simulink model "PubIfDecisionTOS_MDL"  (R2020b)
settings: configuration reference "DspaceConfig" (kept outside this file)
PostLoadFcn:
  | if any(exist('dsrtsu_mdlpostloadfcn', 'file') ~= 0), dsrtsu_mdlpostloadfcn('Execute', bdroot); end
InitFcn:
  | , if any(exist('dsmpb_private', 'file') ~= 0), dsmpb_private('dsmpb_mdlclblib', 'Init', bdroot); end,
undefined symbols (not defined in the file or in its folder): C_TOS_ACCEgoRAxletoFbumplength_m, C_TOS_ACCTargetFront_Flag, C_TOS_AEBJAPedObjDxThre_Val, C_TOS_AEBJAPedObjDyThre_Val, C_TOS_AEBJATargetSize_Val, C_TOS_AEBJAVehObjDxThre_Val, C_TOS_AEBJAVehObjDyThre_Val, C_TOS_AEBJuncPedTargetSize_Val, C_TOS_AEBLatObjDxThre_Val, C_TOS_AEBLatPedDyThre_Val, C_TOS_AEBLatTargetSize_Val, C_TOS_AEBLongTargetInEgoFront_Flag, C_TOS_axAbsGround_Parameter, C_TOS_CameraConfirmedFlag, C_TOS_CNsubjWidth, C_TOS_CurrentLaneCoreMinWidth_Val, C_TOS_CutInProb_Val_Zero, C_TOS_CutOutProb_Val_Zero, C_TOS_D2R_Val, C_TOS_DefaultValueObjectToCenterLine_dy, C_TOS_EgoCarWidth_Val, C_TOS_EgoDxRefPoint_m, C_TOS_EgoRAxletoFbumplength_m, C_TOS_HalfWidthVehicle_Con, C_TOS_HWA_CurrentLaneFlag, C_TOS_HWA_LeftLaneFlag, C_TOS_HWA_MovingDir_Vaild, C_TOS_HWA_MovState_Vaild, C_TOS_HWA_RightLaneFlag, C_TOS_LaneLineCourseErrorFront, C_TOS_LaneLineCourseErrorRear, C_TOS_MotorbikeDefaultWidth_m, C_TOS_NumberOfEffectiveTargets, C_TOS_Obj_Age_Val, C_TOS_Objdx_Constraint_Val, C_TOS_ObjectDefaultWidth_m, C_TOS_ObjInCurrentLane_Val, C_TOS_ObjInCurrentLaneValid, C_TOS_ObjInLeftLaneValid, C_TOS_ObjInRightLaneValid, C_TOS_ObjNotInCurrentLane_Val, C_TOS_ObjNotREElementType, C_TOS_ObjPredictDis_dy_ConstantVal_Zeros, C_TOS_ObjToCenterLine_ConstantVal_Zeros, C_TOS_OFMObjIDInvilad_Val, C_TOS_PIL_LatDisCons_Val_zero, C_TOS_PIL_ObjectCutInFlag_b, C_TOS_PIL_ObjectCutOutFlag_b, C_TOS_PIL_ObjLaneProb_al_Val, C_TOS_PP_ObjFusType_FC_Confirm_b, C_TOS_PP_ObjFusType_FC_FR_Confirm_b, C_TOS_PP_ObjFusType_FR_Confirm_b, C_TOS_RE_80BoolDefault_Val, C_TOS_RE_80Single181Default_Val, C_TOS_RE_80Single255Default_Val, C_TOS_RE_80Uint8Default_Val, C_TOS_RE_D2R, C_TOS_RE_D_180_Val, C_TOS_RE_InvalidObjectID_Val, C_TOS_RE_InvalidTargetChainDir_Val ... (+142)
libraries: simulink x1650, TOS_LIB x361, canfdmsglib x14
(part 34 of 69)

== system PubIfDecisionTOS_MDL/TOS_20201112/TOS_2012080320/PP1128/AAT-AdditionalAttributes/PP_ObjectToCenterLine_dy/PP_EgoVeh_Object_ToCenterLine/PP_ObjectToCenterLine/PP_ObjectToCenterLine_/line05_dy ==
  Object_DX : Inport
  line05_C0 : Inport  Port=2
  line05_C1 : Inport  Port=3
  line05_C2 : Inport  Port=4
  line05_C3 : Inport  Port=5
  Add : Sum
  Add1 : Sum
  Add3 : Sum
  Constant1 : Constant  Value=3  OutDataTypeStr=single
  Math Function1 : Math  Operator=pow  SignedPower=on  SaturateOnIntegerOverflow=on
  Product : Product
  Product1 : Product
  Product2 : Product
  Square : Math  Operator=square  SignedPower=on  SaturateOnIntegerOverflow=on
  line05_dy : Outport
  wires:
  line05_C1/1 -> Product1/2
  line05_C3/1 -> Product2/2
  Add3/1 -> line05_dy/1
  Add/1 -> Add3/1
  Constant1/1 -> Math Function1/2
  Product1/1 -> Add1/2
  Product2/1 -> Add3/2
  Math Function1/1 -> Product2/1
  Object_DX/1 -> Math Function1/1, Square/1, Product1/1
  Square/1 -> Product/1
  line05_C2/1 -> Product/2
  Product/1 -> Add/2
  line05_C0/1 -> Add1/1
  Add1/1 -> Add/1

== system PubIfDecisionTOS_MDL/TOS_20201112/TOS_2012080320/PP1128/AAT-AdditionalAttributes/PP_ObjectToCenterLine_dy/PP_EgoVeh_Object_ToCenterLine/PP_ObjectToCenterLine/PP_ObjectToCenterLine_/line06_DisJudge ==
  Object_DX : Inport
  line06_dDisStart : Inport  Port=2
  line06_dDisEnd : Inport  Port=3
  Logical Operator : Logic  AllPortsSameDT=off  OutDataTypeStr=boolean
  Relational Operator : RelationalOperator  OutDataTypeStr=boolean  RndMeth=Nearest
  Relational Operator1 : RelationalOperator  Operator=<  OutDataTypeStr=boolean  RndMeth=Nearest
  line06_DisJudge : Outport
  wires:
  Logical Operator/1 -> line06_DisJudge/1
  Relational Operator1/1 -> Logical Operator/2
  Relational Operator/1 -> Logical Operator/1
  Object_DX/1 -> Relational Operator/1, Relational Operator1/1
  line06_dDisStart/1 -> Relational Operator/2
  line06_dDisEnd/1 -> Relational Operator1/2

== system PubIfDecisionTOS_MDL/TOS_20201112/TOS_2012080320/PP1128/AAT-AdditionalAttributes/PP_ObjectToCenterLine_dy/PP_EgoVeh_Object_ToCenterLine/PP_ObjectToCenterLine/PP_ObjectToCenterLine_/line06_dy ==
  Object_DX : Inport
  line06_C0 : Inport  Port=2
  line06_C1 : Inport  Port=3
  line06_C2 : Inport  Port=4
  line6_C3 : Inport  Port=5
  Add : Sum
  Add1 : Sum
  Add3 : Sum
  Constant1 : Constant  Value=3  OutDataTypeStr=single
  Math Function1 : Math  Operator=pow  SignedPower=on  SaturateOnIntegerOverflow=on
  Product : Product
  Product1 : Product
  Product2 : Product
  Square : Math  Operator=square  SignedPower=on  SaturateOnIntegerOverflow=on
  line6_dy : Outport
  wires:
  Add1/1 -> Add/1
  line06_C0/1 -> Add1/1
  Product/1 -> Add/2
  line06_C2/1 -> Product/2
  Square/1 -> Product/1
  Object_DX/1 -> Product1/1, Square/1, Math Function1/1
  Math Function1/1 -> Product2/1
  Product2/1 -> Add3/2
  Product1/1 -> Add1/2
  Constant1/1 -> Math Function1/2
  Add/1 -> Add3/1
  Add3/1 -> line6_dy/1
  line6_C3/1 -> Product2/2
  line06_C1/1 -> Product1/2

== system PubIfDecisionTOS_MDL/TOS_20201112/TOS_2012080320/PP1128/AAT-AdditionalAttributes/PP_ObjectToCenterLine_dy/PP_ObjectToCenterLine_vyc/PP_ObjectToCenterLine_vyc_Filt/ObjectToCenterLine_vyc/ObjectToCenterLine_vyc_Filt ==
  ObjectID_Filt_K1 : Inport
  PP_ObjectToCenterLine_vyc_Filt_K1 : Inport  Port=2  OutDataTypeStr=single
  PP_ObjectToCenterLine_vyc : Inport  Port=3  OutDataTypeStr=single
  Object_ID : Inport  Port=4  OutDataTypeStr=uint8
  Object_Age : Inport  Port=5
  TOS_OFMObjValid_Flag : Inport  Port=6
  Action Port : ActionPort  ActionPortLabel=else
  Constant1 : Constant  Value=C_TOS_NumberOfEffectiveTargets  OutDataTypeStr=int32
      settings: AttributesFormatString=C_TOS_NumberOfEffectiveTargets = 80
  Constant2 : Constant  Value=0.2  OutDataTypeStr=single
      settings: AttributesFormatString=P_TOS_PIL_ObjectToCenterLine_dy_CutInDeclineLimit = 0.1
  Constant8 : Constant  Value=0.35  OutDataTypeStr=single
      settings: AttributesFormatString=P_TOS_PIL_ObjectToCenterLine_dy_CutInUpperLimit = 0.5
  ObjectToCenterLine_vyc_Filt : MATLAB Function  TreatAsAtomicUnit=on
  Terminator : Terminator
  Obj_ID : Outport
  PP_ObjectToCenterLine_vyc_Filt : Outport  Port=2  OutDataTypeStr=single
  wires:
  TOS_OFMObjValid_Flag/1 -> ObjectToCenterLine_vyc_Filt/5(TOS_OFMObjValid_Flag)
  Object_Age/1 -> Terminator/1
  PP_ObjectToCenterLine_vyc_Filt_K1/1 -> ObjectToCenterLine_vyc_Filt/2(ObjectToCenterLine_dy_Filt_K1)
  Object_ID/1 -> Obj_ID/1, ObjectToCenterLine_vyc_Filt/4(Object_ID)
  ObjectID_Filt_K1/1 -> ObjectToCenterLine_vyc_Filt/1(ObjectID_Filt_K1)
  Constant2/1 -> ObjectToCenterLine_vyc_Filt/7(P_TOS_PIL_ObjectToCenterLine_dy_CutInDeclineLimit)
  Constant1/1 -> ObjectToCenterLine_vyc_Filt/8(Iterator_Num)
  PP_ObjectToCenterLine_vyc/1 -> ObjectToCenterLine_vyc_Filt/3(ObjectToCenterLine_dy)
  Constant8/1 -> ObjectToCenterLine_vyc_Filt/6(P_TOS_PIL_ObjectToCenterLine_dy_CutInUpperLimit)
  ObjectToCenterLine_vyc_Filt/1(ObjectToCenterLine_dy_Filt) -> PP_ObjectToCenterLine_vyc_Filt/1

== system PubIfDecisionTOS_MDL/TOS_20201112/TOS_2012080320/PP1128/AAT-AdditionalAttributes/PP_ObjectToCenterLine_dy/PP_ObjectToCenterLine_vyc/PP_ObjectToCenterLine_vyc_Filt/ObjectToCenterLine_vyc/ObjectToCenterLine_vyc_FiltDefault ==
  Action Port : ActionPort  ActionPortLabel=if(u1 ~= 0)
  Constant : Constant  Value=0  OutDataTypeStr=uint8
  Constant1 : Constant  Value=255  OutDataTypeStr=single
  Obj_ID : Outport
  ObjectToCenterLine_dy_Filt : Outport  Port=2  OutDataTypeStr=single
  wires:
  Constant1/1 -> ObjectToCenterLine_dy_Filt/1
  Constant/1 -> Obj_ID/1

== system PubIfDecisionTOS_MDL/TOS_20201112/TOS_2012080320/PP1128/AAT-AdditionalAttributes/RoadEdge/RE_2020_12_07/RoadEdge_V2/RoadEdgeElementFinalJudge/EgoLeft_RoadEdgeElementsFinalJudge ==
  RE_EgoLeftEdgeGroupChainElementCount : Inport  OutDataTypeStr=uint8  BusOutputAsStruct=on
  RE_EgoLeft_3TargetTheta : Inport  Port=2  OutDataTypeStr=single  BusOutputAsStruct=on
  RE_EgoLeft_2TargetTheta : Inport  Port=3  OutDataTypeStr=single  BusOutputAsStruct=on
  RE_EgoLeft_StillObjSortIndex : Inport  Port=4  OutDataTypeStr=uint8  BusOutputAsStruct=on
  vxvRefMs : Inport  Port=5  OutDataTypeStr=single  PortDimensions=1  BusOutputAsStruct=on
  Object_Dx : Inport  Port=6  OutDataTypeStr=single  BusOutputAsStruct=on
  Object_Dy : Inport  Port=7  OutDataTypeStr=single  BusOutputAsStruct=on
  Object_ID : Inport  Port=8  OutDataTypeStr=uint8  BusOutputAsStruct=on
  RE_EdgeElementID_K1 : Inport  Port=9
  Dy_Filter : Subsystem
  For Each Subsystem : Subsystem  TreatAsAtomicUnit=on
  RoadEdgeElementFinalJudge : Stateflow chart  TreatAsAtomicUnit=on
  Unit Delay{,1..3} (4 alike) : UnitDelay  SampleTime=-1  HasFrameUpgradeWarning=on
  RE_EgoLeftEdgeElementFlag : Outport
  RE_EgoLeftEdgeElementType : Outport  Port=2
  StillTarget34_13_Theta_ALL : Outport  Port=3
  RE_EgoLeftEdgeElementID : Outport  Port=4
  EdgeGroupChainElementCount_OFM : Outport  Port=5
  wires:
  RE_EgoLeftEdgeGroupChainElementCount/1 -> RoadEdgeElementFinalJudge/2(EdgeGroupChainElementCount)
  RE_EgoLeft_3TargetTheta/1 -> RoadEdgeElementFinalJudge/3(RE_3TargetTheta)
  RE_EgoLeft_2TargetTheta/1 -> RoadEdgeElementFinalJudge/4(RE_2TargetTheta)
  RE_EgoLeft_StillObjSortIndex/1 -> RoadEdgeElementFinalJudge/5(RE_StillObjectSortIndex), Unit Delay2/1
  Object_Dx/1 -> RoadEdgeElementFinalJudge/8(Object_Dx)
  vxvRefMs/1 -> RoadEdgeElementFinalJudge/7(Ego_Vxv)
  Object_ID/1 -> Dy_Filter/4(Object_ID), RoadEdgeElementFinalJudge/10(Object_ID)
  RoadEdgeElementFinalJudge/1(RoadEdgeElementFlag) -> Unit Delay/1, RE_EgoLeftEdgeElementFlag/1  "EdgeElementFlag"
  RoadEdgeElementFinalJudge/2(RE_EdgeElementType) -> RE_EgoLeftEdgeElementType/1  "EdgeElementType"
  RoadEdgeElementFinalJudge/3(StillTarget34_13_Theta_ALL) -> StillTarget34_13_Theta_ALL/1  "StillTarget34_13_Theta_ALL"
  RoadEdgeElementFinalJudge/4(RE_EdgeElementID) -> RE_EgoLeftEdgeElementID/1  "RE_EgoLeftEdgeElementID"
  RoadEdgeElementFinalJudge/5(StillTarget13_Theta_ALL) -> Unit Delay1/1
  Unit Delay1/1 -> RoadEdgeElementFinalJudge/11(RE_13TargetTheta_ALL)
  Unit Delay2/1 -> RoadEdgeElementFinalJudge/6(RE_StillObjectSortIndex_K1)
  Object_Dy/1 -> Dy_Filter/1(Object_Dy), Unit Delay3/1
  Unit Delay3/1 -> Dy_Filter/2(Object_Dy_K1)
  Dy_Filter/1(Object_DyFilter) -> RoadEdgeElementFinalJudge/9(Object_Dy)
  For Each Subsystem/1(RE_4StepEdgeElementFlag) -> RoadEdgeElementFinalJudge/1(RE_4StepEdgeElementFlag)
  Unit Delay/1 -> For Each Subsystem/1(RE_EdgeElementFlag)
  RoadEdgeElementFinalJudge/10(EdgeGroupChainElementCount_OFM) -> EdgeGroupChainElementCount_OFM/1
  RE_EdgeElementID_K1/1 -> Dy_Filter/3(RE_EdgeElementID_K1)

== system PubIfDecisionTOS_MDL/TOS_20201112/TOS_2012080320/PP1128/AAT-AdditionalAttributes/RoadEdge/RE_2020_12_07/RoadEdge_V2/RoadEdgeElementFinalJudge/EgoRight_RoadEdgeElementsFinalJudge ==
  note: 13_Theta
  note: StillTarget34_13_Theta_ALL
  note: StillObjSortIndex
  note: 2TargetTheta
  note: 3TargetTheta
  note: RE_EgoRightEdgeGroupChainElementCount
  note: StillTarget13_Theta_OFM
  note: StillTarget34_13_Theta_OFM
  note: RE_EdgeElementID
  note: StillTarget3Theta_OFM
  note: StillTarget2Theta_OFM
  RE_EgoRightEdgeGroupChainElementCount : Inport  OutDataTypeStr=uint8  BusOutputAsStruct=on
  RE_EgoRight_3TargetTheta : Inport  Port=2  OutDataTypeStr=single  BusOutputAsStruct=on
  RE_EgoRight_2TargetTheta : Inport  Port=3  OutDataTypeStr=single  BusOutputAsStruct=on
  RE_EgoRight_StillObjSortIndex : Inport  Port=4  OutDataTypeStr=uint8  BusOutputAsStruct=on
  vxvRefMs : Inport  Port=5  OutDataTypeStr=single  PortDimensions=1  BusOutputAsStruct=on
  Object_Dx : Inport  Port=6  OutDataTypeStr=single  BusOutputAsStruct=on
  Object_Dy : Inport  Port=7  OutDataTypeStr=single  BusOutputAsStruct=on
  Object_ID : Inport  Port=8  OutDataTypeStr=uint8  BusOutputAsStruct=on
  RE_EdgeElementID_K1 : Inport  Port=9
  Display{1..12} (12 alike) : Display
  Dy_Filter : Subsystem
  For Each Subsystem : Subsystem  TreatAsAtomicUnit=on
  RoadEdgeElementFinalJudge : Stateflow chart  TreatAsAtomicUnit=on
  Unit Delay{,1..3} (4 alike) : UnitDelay  SampleTime=-1  HasFrameUpgradeWarning=on
  RE_EgoRightEdgeElementFlag : Outport
  RE_EgoRightEdgeElementType : Outport  Port=2
  StillTarget34_13_Theta_ALL : Outport  Port=3
  RE_EgoRightEdgeElementID : Outport  Port=4
  EdgeGroupChainElementCount_OFM : Outport  Port=5
  wires:
  Unit Delay/1 -> For Each Subsystem/1(RE_EdgeElementFlag)
  For Each Subsystem/1(RE_4StepEdgeElementFlag) -> RoadEdgeElementFinalJudge/1(RE_4StepEdgeElementFlag)
  RoadEdgeElementFinalJudge/9(StillTarget2Theta_OFM) -> Display5/1  "StillTarget2Theta_OFM"
  RoadEdgeElementFinalJudge/8(StillTarget3Theta_OFM) -> Display4/1  "StillTarget3Theta_OFM"
  RoadEdgeElementFinalJudge/7(StillTarget34_13_Theta_OFM) -> Display2/1  "StillTarget13_Theta"
  RoadEdgeElementFinalJudge/6(StillTarget13_Theta_OFM) -> Display1/1  "StillTarget13_Theta_OFM"
  Dy_Filter/1(Object_DyFilter) -> RoadEdgeElementFinalJudge/9(Object_Dy)
  Object_Dy/1 -> Unit Delay3/1, Dy_Filter/1(Object_Dy)
  Unit Delay2/1 -> RoadEdgeElementFinalJudge/6(RE_StillObjectSortIndex_K1)
  Unit Delay1/1 -> RoadEdgeElementFinalJudge/11(RE_13TargetTheta_ALL)
  RoadEdgeElementFinalJudge/5(StillTarget13_Theta_ALL) -> Display11/1, Unit Delay1/1
  RoadEdgeElementFinalJudge/4(RE_EdgeElementID) -> Display3/1, RE_EgoRightEdgeElementID/1
  RoadEdgeElementFinalJudge/3(StillTarget34_13_Theta_ALL) -> Display10/1, StillTarget34_13_Theta_ALL/1  "StillTarget34_13_Theta_ALL"
  RoadEdgeElementFinalJudge/2(RE_EdgeElementType) -> RE_EgoRightEdgeElementType/1  "EdgeElementType"
  RoadEdgeElementFinalJudge/1(RoadEdgeElementFlag) -> Unit Delay/1, RE_EgoRightEdgeElementFlag/1  "EdgeElementFlag"
  Object_ID/1 -> RoadEdgeElementFinalJudge/10(Object_ID), Dy_Filter/4(Object_ID)
  vxvRefMs/1 -> RoadEdgeElementFinalJudge/7(Ego_Vxv)
  Object_Dx/1 -> RoadEdgeElementFinalJudge/8(Object_Dx)
  RE_EgoRight_StillObjSortIndex/1 -> RoadEdgeElementFinalJudge/5(RE_StillObjectSortIndex), Display6/1, Unit Delay2/1
  RE_EgoRight_2TargetTheta/1 -> RoadEdgeElementFinalJudge/4(RE_2TargetTheta), Display7/1
  RE_EgoRight_3TargetTheta/1 -> RoadEdgeElementFinalJudge/3(RE_3TargetTheta), Display8/1
  RE_EgoRightEdgeGroupChainElementCount/1 -> RoadEdgeElementFinalJudge/2(EdgeGroupChainElementCount), Display9/1
  RoadEdgeElementFinalJudge/10(EdgeGroupChainElementCount_OFM) -> Display12/1, EdgeGroupChainElementCount_OFM/1
  RE_EdgeElementID_K1/1 -> Dy_Filter/3(RE_EdgeElementID_K1)
  Unit Delay3/1 -> Dy_Filter/2(Object_Dy_K1)

== system PubIfDecisionTOS_MDL/TOS_20201112/TOS_2012080320/PP1128/AAT-AdditionalAttributes/RoadEdge/RE_2020_12_07/RoadEdge_V2/RoadEdgeElementType/Chart/FinalConfirm.FusType ==
  ObjectFusType : Inport  OutDataTypeStr=uint8  PortDimensions=1
  f : TriggerPort  TriggerType=function-call  VariantControl=(inherit)
      settings: CopyFcn=Stateflow.SLINSF.SimulinkMan.removeBlockPreDeleteFcn  PreDeleteFcn=Stateflow.SLINSF.SimulinkMan.unsafePredeleteFcn
  Data Type Conversion1 : DataTypeConversion  OutDataTypeStr=Enum: OFM_OBJ_FUSTYPE
  Enumerated Constant63 : simulink/Sources/Enumerated Constant  OutDataTypeStr=Enum: OFM_OBJ_FUSTYPE  Value=OFM_OBJ_FUSTYPE.FR  SampleTime=inf
      settings: AttributesFormatString=OFM_OBJ_FUSTYPE.FR = 2
  Enumerated Constant65 : simulink/Sources/Enumerated Constant  OutDataTypeStr=Enum: OFM_OBJ_FUSTYPE  Value=OFM_OBJ_FUSTYPE.FR_CL  SampleTime=inf
      settings: AttributesFormatString=OFM_OBJ_FUSTYPE.FR_CL = 6
  Enumerated Constant67 : simulink/Sources/Enumerated Constant  OutDataTypeStr=Enum: OFM_OBJ_FUSTYPE  Value=OFM_OBJ_FUSTYPE.FR_CR  SampleTime=inf
      settings: AttributesFormatString=OFM_OBJ_FUSTYPE.FR_CR = 10
  Enumerated Constant69 : simulink/Sources/Enumerated Constant  OutDataTypeStr=Enum: OFM_OBJ_FUSTYPE  Value=OFM_OBJ_FUSTYPE.FR_CL_CR  SampleTime=inf
      settings: AttributesFormatString=OFM_OBJ_FUSTYPE.FR_CL_CR = 14
  Enumerated Constant71 : simulink/Sources/Enumerated Constant  OutDataTypeStr=Enum: OFM_OBJ_FUSTYPE  Value=OFM_OBJ_FUSTYPE.FR_BL  SampleTime=inf
      settings: AttributesFormatString=OFM_OBJ_FUSTYPE.FR_BL = 18
  Enumerated Constant73 : simulink/Sources/Enumerated Constant  OutDataTypeStr=Enum: OFM_OBJ_FUSTYPE  Value=OFM_OBJ_FUSTYPE.FR_CL_BL  SampleTime=inf
      settings: AttributesFormatString=OFM_OBJ_FUSTYPE.FR_CL_BL = 22
  Enumerated Constant75 : simulink/Sources/Enumerated Constant  OutDataTypeStr=Enum: OFM_OBJ_FUSTYPE  Value=OFM_OBJ_FUSTYPE.FR_CR_BL  SampleTime=inf
      settings: AttributesFormatString=OFM_OBJ_FUSTYPE.FR_CR_BL = 26
  Enumerated Constant77 : simulink/Sources/Enumerated Constant  OutDataTypeStr=Enum: OFM_OBJ_FUSTYPE  Value=OFM_OBJ_FUSTYPE.FR_CL_CR_BL  SampleTime=inf
      settings: AttributesFormatString=OFM_OBJ_FUSTYPE.FR_CL_CR_BL = 30
  Enumerated Constant79 : simulink/Sources/Enumerated Constant  OutDataTypeStr=Enum: OFM_OBJ_FUSTYPE  Value=OFM_OBJ_FUSTYPE.FR_BR  SampleTime=inf
      settings: AttributesFormatString=OFM_OBJ_FUSTYPE.FR_BR = 34
  Enumerated Constant81 : simulink/Sources/Enumerated Constant  OutDataTypeStr=Enum: OFM_OBJ_FUSTYPE  Value=OFM_OBJ_FUSTYPE.FR_CL_BR  SampleTime=inf
      settings: AttributesFormatString=OFM_OBJ_FUSTYPE.FR_CL_BR = 38
  Enumerated Constant83 : simulink/Sources/Enumerated Constant  OutDataTypeStr=Enum: OFM_OBJ_FUSTYPE  Value=OFM_OBJ_FUSTYPE.FR_CR_BR  SampleTime=inf
      settings: AttributesFormatString=OFM_OBJ_FUSTYPE.FR_CR_BR = 42
  Enumerated Constant85 : simulink/Sources/Enumerated Constant  OutDataTypeStr=Enum: OFM_OBJ_FUSTYPE  Value=OFM_OBJ_FUSTYPE.FR_CL_CR_BR  SampleTime=inf
      settings: AttributesFormatString=OFM_OBJ_FUSTYPE.FR_CL_CR_BR = 46
  Enumerated Constant87 : simulink/Sources/Enumerated Constant  OutDataTypeStr=Enum: OFM_OBJ_FUSTYPE  Value=OFM_OBJ_FUSTYPE.FR_BL_BR  SampleTime=inf
      settings: AttributesFormatString=OFM_OBJ_FUSTYPE.FR_BL_BR = 50
  Enumerated Constant89 : simulink/Sources/Enumerated Constant  OutDataTypeStr=Enum: OFM_OBJ_FUSTYPE  Value=OFM_OBJ_FUSTYPE.FR_CL_BL_BR  SampleTime=inf
      settings: AttributesFormatString=OFM_OBJ_FUSTYPE.FR_CL_BL_BR = 54
  Enumerated Constant91 : simulink/Sources/Enumerated Constant  OutDataTypeStr=Enum: OFM_OBJ_FUSTYPE  Value=OFM_OBJ_FUSTYPE.FR_CR_BL_BR  SampleTime=inf
      settings: AttributesFormatString=OFM_OBJ_FUSTYPE.FR_CR_BL_BR = 58
  Enumerated Constant93 : simulink/Sources/Enumerated Constant  OutDataTypeStr=Enum: OFM_OBJ_FUSTYPE  Value=OFM_OBJ_FUSTYPE.FR_CL_CR_BL_BR  SampleTime=inf
      settings: AttributesFormatString=OFM_OBJ_FUSTYPE.FR_CL_CR_BL_BR = 62
  Logical Operator15 : Logic  Operator=OR  Inputs=16  AllPortsSameDT=off  OutDataTypeStr=boolean
  Relational Operator{16,20,22,24,26,28,30,32,34,36,38,40,42,44,46,48} (16 alike) : RelationalOperator  Operator===  OutDataTypeStr=boolean  RndMeth=Nearest
  RE_Object_FR_Other : Outport
  wires:
  Enumerated Constant67/1 -> Relational Operator22/2
  Enumerated Constant91/1 -> Relational Operator46/2
  Enumerated Constant87/1 -> Relational Operator42/2
  Enumerated Constant63/1 -> Relational Operator16/2
  Relational Operator36/1 -> Logical Operator15/10
  Enumerated Constant65/1 -> Relational Operator20/2
  Relational Operator46/1 -> Logical Operator15/15
  Enumerated Constant83/1 -> Relational Operator38/2
  Relational Operator42/1 -> Logical Operator15/13
  Relational Operator44/1 -> Logical Operator15/14
  Relational Operator32/1 -> Logical Operator15/8
  Enumerated Constant77/1 -> Relational Operator32/2
  ObjectFusType/1 -> Data Type Conversion1/1
  Relational Operator40/1 -> Logical Operator15/12
  Enumerated Constant93/1 -> Relational Operator48/2
  Logical Operator15/1 -> RE_Object_FR_Other/1
  Enumerated Constant89/1 -> Relational Operator44/2
  Relational Operator38/1 -> Logical Operator15/11
  Relational Operator48/1 -> Logical Operator15/16
  Relational Operator28/1 -> Logical Operator15/6
  Relational Operator20/1 -> Logical Operator15/2
  Relational Operator24/1 -> Logical Operator15/4
  Enumerated Constant73/1 -> Relational Operator28/2
  Relational Operator30/1 -> Logical Operator15/7
  Enumerated Constant81/1 -> Relational Operator36/2
  Enumerated Constant85/1 -> Relational Operator40/2
  Enumerated Constant71/1 -> Relational Operator26/2
  Relational Operator34/1 -> Logical Operator15/9
  Enumerated Constant69/1 -> Relational Operator24/2
  Enumerated Constant75/1 -> Relational Operator30/2
  Enumerated Constant79/1 -> Relational Operator34/2
  Relational Operator16/1 -> Logical Operator15/1
  Relational Operator26/1 -> Logical Operator15/5
  Relational Operator22/1 -> Logical Operator15/3
  Data Type Conversion1/1 -> Relational Operator20/1, Relational Operator22/1, Relational Operator24/1, Relational Operator26/1, Relational Operator28/1, Relational Operator30/1, Relational Operator32/1, Relational Operator34/1, Relational Operator36/1, Relational Operator38/1, Relational Operator40/1, Relational Operator42/1, Relational Operator44/1, Relational Operator46/1, Relational Operator48/1, Relational Operator16/1

== system PubIfDecisionTOS_MDL/TOS_20201112/TOS_2012080320/PP1128/AAT-AdditionalAttributes/RoadEdge/RE_2020_12_07/RoadEdge_V2/RoadEdgeElementType/For Each Subsystem ==
  EdgeElementID : Inport  Partition=on  PartitionDimension=1  PartitionWidth=1  PartitionOffset=0
  EdgeElementID_K1 : Inport  Port=2  Partition=on  PartitionDimension=1  PartitionWidth=1  PartitionOffset=0
  Constant : Constant  Value=P_TOS_RE_stateProlongationTime  OutDataTypeStr=single
      settings: AttributesFormatString=%<Value> = 0.2
  Constant1 : Constant  Value=P_TOS_RE_Ts  OutDataTypeStr=single
      settings: AttributesFormatString=%<Value> = 0.05
  For Each : ForEach  DisableCoverage=on
  StateDelayAbortion : Stateflow chart  TreatAsAtomicUnit=on
  Terminator : Terminator
  RE_EdgeElementID : Outport  ConcatenationDimension=1
  wires:
  StateDelayAbortion/2(stateOut) -> RE_EdgeElementID/1
  EdgeElementID/1 -> StateDelayAbortion/1(state)
  StateDelayAbortion/1(timeSinceLastState) -> Terminator/1
  Constant/1 -> StateDelayAbortion/3(stateProlongationTime)
  Constant1/1 -> StateDelayAbortion/4(Ts)
  EdgeElementID_K1/1 -> StateDelayAbortion/2(stateK1)

== system PubIfDecisionTOS_MDL/TOS_20201112/TOS_2012080320/PP1128/AAT-AdditionalAttributes/RoadEdge/RE_2020_12_07/RoadEdge_V2/RoadEdgeElementType/For Each Subsystem1 ==
  EdgeElementType : Inport  Partition=on  PartitionDimension=1  PartitionWidth=1  PartitionOffset=0
  EdgeElementType_K1 : Inport  Port=2  Partition=on  PartitionDimension=1  PartitionWidth=1  PartitionOffset=0
  Constant : Constant  Value=P_TOS_RE_stateProlongationTime  OutDataTypeStr=single
      settings: AttributesFormatString=%<Value> = 0.2
  Constant1 : Constant  Value=P_TOS_RE_Ts  OutDataTypeStr=single
      settings: AttributesFormatString=%<Value> = 0.05
  For Each : ForEach  DisableCoverage=on
  StateDelayAbortion : Stateflow chart  TreatAsAtomicUnit=on
  Terminator : Terminator
  RE_EdgeElementType : Outport  ConcatenationDimension=1
  wires:
  EdgeElementType_K1/1 -> StateDelayAbortion/2(stateK1)
  Constant1/1 -> StateDelayAbortion/4(Ts)
  Constant/1 -> StateDelayAbortion/3(stateProlongationTime)
  StateDelayAbortion/1(timeSinceLastState) -> Terminator/1
  EdgeElementType/1 -> StateDelayAbortion/1(state)
  StateDelayAbortion/2(stateOut) -> RE_EdgeElementType/1

== system PubIfDecisionTOS_MDL/TOS_20201112/TOS_2012080320/PP1128/AAT-AdditionalAttributes/RoadEdge/RE_2020_12_07/RoadEdge_V2/SelectStationaryObjects/SelectStationaryObject ==
  note: 筛选符合如下条件目标：
      | [1]FR_Other
      | [2] fus.object.stand_b = True;
      | [3]-100m<dx<200m;
      | [4]-20m<dy<20m;
      | [5]dxv 的方差小于 12.5 ；
      | [6]dyv 的方差小于 12.5;
  Object_ID : Inport  Partition=on  PartitionDimension=1  PartitionWidth=1  PartitionOffset=0
  Object_FusType : Inport  Port=2  Partition=on  PartitionDimension=1  PartitionWidth=1  PartitionOffset=0
  Object_MovingState : Inport  Port=3  Partition=on  PartitionDimension=1  PartitionWidth=1  PartitionOffset=0
  Object_Dx : Inport  Port=4  Partition=on  PartitionDimension=1  PartitionWidth=1  PartitionOffset=0
  Object_Dy : Inport  Port=5  Partition=on  PartitionDimension=1  PartitionWidth=1  PartitionOffset=0
  Object_DxStd : Inport  Port=6  Partition=on  PartitionDimension=1  PartitionWidth=1  PartitionOffset=0
  Object_DyStd : Inport  Port=7  Partition=on  PartitionDimension=1  PartitionWidth=1  PartitionOffset=0
  Object_ExistProb : Inport  Port=8  Partition=on  PartitionDimension=1  PartitionWidth=1  PartitionOffset=0
  Object_ExistProb_K1 : Inport  Port=9  Partition=on  PartitionDimension=1  PartitionWidth=1  PartitionOffset=0
  Compare To Constant : simulink/Logic and Bit Operations/Compare To Constant  relop===  const=C_TOS_RE_InvalidObjectID_Val  OutDataTypeStr=boolean
      settings: AttributesFormatString=%<const> = 0
  For Each : ForEach  DisableCoverage=on
  If : If  IfExpression=u1
  Merge : Merge
  RE_StationaryObjectsSortCond : Subsystem  TreatAsAtomicUnit=on
  RE_StationaryObjectsSortDefault : Subsystem  TreatAsAtomicUnit=on
  RE_StationaryObjectFlag : Outport  ConcatenationDimension=1
  wires:
  Compare To Constant/1 -> If/1
  If/2 -> RE_StationaryObjectsSortCond/Action
  If/1 -> RE_StationaryObjectsSortDefault/Action
  RE_StationaryObjectsSortCond/1(RE_StationaryObjectFlag) -> Merge/2
  RE_StationaryObjectsSortDefault/1(RE_StationaryObjectFlag) -> Merge/1
  Merge/1 -> RE_StationaryObjectFlag/1
  Object_ID/1 -> Compare To Constant/1
  Object_FusType/1 -> RE_StationaryObjectsSortCond/1(Object_FusType)
  Object_MovingState/1 -> RE_StationaryObjectsSortCond/2(Object_MovingState)
  Object_Dx/1 -> RE_StationaryObjectsSortCond/3(Object_Dx)
  Object_Dy/1 -> RE_StationaryObjectsSortCond/4(Object_Dy)
  Object_DxStd/1 -> RE_StationaryObjectsSortCond/5(Object_DxStd)
  Object_DyStd/1 -> RE_StationaryObjectsSortCond/6(Object_DyStd)
  Object_ExistProb/1 -> RE_StationaryObjectsSortCond/7(Object_ExistProb)
  Object_ExistProb_K1/1 -> RE_StationaryObjectsSortCond/8(Object_ExistProb_K1)

== system PubIfDecisionTOS_MDL/TOS_20201112/TOS_2012080320/PP1128/AAT-AdditionalAttributes/RoadEdge/RE_2020_12_07/RoadEdge_V2/TargetChain/EgoLeftTargetChainDirection ==
  note: RE_TargetChainStartDir:
      |
      | 0:Invalid
      | 1:Stright Dir
      | 2:Left Dir
      | 3:Right Dir
  note: RE_TargetChainDir:
      |
      | 0:Invalid
      | 1:Stright_Same Dir
      | 2:Stright_Different Dir
      | 3:Left_Same Dir
      | 4:Left_Different Dir
      | 5:Right_Same Dir
      | 6:Right_Different Dir
  note: 判断目标链的方向；直向/左向/右向
      | 同向/异向
  note: 按Dx从小到大顺序提取目标；
      | 计算与上一个目标连线的斜率角
  RE_EgoLeftStationaryObjectsSortIndex : Inport
  Object_Dx : Inport  Port=2  PortDimensions=80  BusOutputAsStruct=on
  Object_Dy : Inport  Port=3  PortDimensions=80  BusOutputAsStruct=on
  Object_ID : Inport  Port=4
  RE_EdgeElementID_K1 : Inport  Port=5
  Dy_Filter : Subsystem
  TargetChainDirectionCalCulat : Stateflow chart  TreatAsAtomicUnit=on
  Theta_Calculation : Stateflow chart  TreatAsAtomicUnit=on
  Unit Delay : UnitDelay  SampleTime=-1  HasFrameUpgradeWarning=on
  Unit Delay1 : UnitDelay  InitialCondition=181  SampleTime=-1  HasFrameUpgradeWarning=on
  Unit Delay2 : UnitDelay  SampleTime=-1  HasFrameUpgradeWarning=on
  RE_EgoLeftTargetChainStartDirection : Outport
  RE_EgoLeftTargetChainDirection : Outport  Port=2
  RE_EgoLeft3TargetTheta : Outport  Port=3
  RE_EgoLeft2TargetTheta : Outport  Port=4
  wires:
  Object_Dy/1 -> Dy_Filter/1(Object_Dy), Unit Delay2/1
  Object_Dx/1 -> Theta_Calculation/3(Object_Dx)
  Theta_Calculation/2(StillTarget12_0_Theta_ALL) -> RE_EgoLeft2TargetTheta/1, Unit Delay1/1
  TargetChainDirectionCalCulat/1(RE_TargetChainStartDir) -> RE_EgoLeftTargetChainStartDirection/1
  Theta_Calculation/1(StillTarget23_12_Theta_ALL) -> RE_EgoLeft3TargetTheta/1, TargetChainDirectionCalCulat/2(RE_StillTarget_Theta2_ALL)
  RE_EgoLeftStationaryObjectsSortIndex/1 -> Unit Delay/1, Theta_Calculation/1(RE_StationaryObjectsSortIndex), TargetChainDirectionCalCulat/1(RE_StationaryObjectsSortIndex)
  TargetChainDirectionCalCulat/2(RE_TargetChainDir) -> RE_EgoLeftTargetChainDirection/1
  Unit Delay/1 -> Theta_Calculation/2(RE_StationaryObjectsSortIndex_K1)  "RE_StationaryObjectsSortIndex_K1"
  Unit Delay1/1 -> Theta_Calculation/5(RE_2TargetTheta_ALL_K1)
  Dy_Filter/1(Object_DyFilter) -> Theta_Calculation/4(Object_Dy)  "EgoLeftObject_DyFilter"
  Unit Delay2/1 -> Dy_Filter/2(Object_Dy_K1)  "Object_Dy_K1"
  Object_ID/1 -> Dy_Filter/3(Object_ID)
  RE_EdgeElementID_K1/1 -> Dy_Filter/4(RE_EdgeElementID_K1)

== system PubIfDecisionTOS_MDL/TOS_20201112/TOS_2012080320/PP1128/AAT-AdditionalAttributes/RoadEdge/RE_2020_12_07/RoadEdge_V2/TargetChain/EgoRightTargetChainDirection ==
  note: RE_TargetChainStartDir:
      |
      | 0:Invalid
      | 1:Stright Dir
      | 2:Left Dir
      | 3:Right Dir
  note: RE_TargetChainDir:
      |
      | 0:Invalid
      | 1:Stright_Same Dir
      | 2:Stright_Different Dir
      | 3:Left_Same Dir
      | 4:Left_Different Dir
      | 5:Right_Same Dir
      | 6:Right_Different Dir
  note: 判断目标链的方向；直向/左向/右向
      | 同向/异向
  note: 按Dx从小到大顺序提取目标；
      | 计算与上一个目标连线的斜率角
  RE_EgoRightStationaryObjectsSortIndex : Inport
  Object_Dx : Inport  Port=2  PortDimensions=80  BusOutputAsStruct=on
  Object_Dy : Inport  Port=3  PortDimensions=80  BusOutputAsStruct=on
  Object_ID : Inport  Port=4
  RE_EdgeElementID_K1 : Inport  Port=5
  Dy_Filter : Subsystem
  TargetChainDirectionCalCulat : Stateflow chart  TreatAsAtomicUnit=on
  Theta_Calculation : Stateflow chart  TreatAsAtomicUnit=on
  Unit Delay : UnitDelay  SampleTime=-1  HasFrameUpgradeWarning=on
  Unit Delay1 : UnitDelay  InitialCondition=181  SampleTime=-1  HasFrameUpgradeWarning=on
  Unit Delay2 : UnitDelay  SampleTime=-1  HasFrameUpgradeWarning=on
  RE_EgoRightTargetChainStartDirection : Outport
  RE_EgoRightTargetChainDirection : Outport  Port=2
  RE_EgoRight3TargetTheta : Outport  Port=3
  RE_EgoRight2TargetTheta : Outport  Port=4
  wires:
  Object_Dy/1 -> Dy_Filter/1(Object_Dy), Unit Delay2/1
  Unit Delay2/1 -> Dy_Filter/2(Object_Dy_K1)  "Object_Dy_K1"
  Dy_Filter/1(Object_DyFilter) -> Theta_Calculation/4(Object_Dy)  "EgoRightObject_DyFilter"
  Unit Delay1/1 -> Theta_Calculation/5(RE_2TargetTheta_ALL_K1)
  Unit Delay/1 -> Theta_Calculation/2(RE_StationaryObjectsSortIndex_K1)  "RE_StationaryObjectsSortIndex_K1"
  Object_ID/1 -> Dy_Filter/3(Object_ID)
  Object_Dx/1 -> Theta_Calculation/3(Object_Dx)
  Theta_Calculation/1(StillTarget23_12_Theta_ALL) -> TargetChainDirectionCalCulat/2(RE_StillTarget_Theta2_ALL), RE_EgoRight3TargetTheta/1
  RE_EgoRightStationaryObjectsSortIndex/1 -> Unit Delay/1, Theta_Calculation/1(RE_StationaryObjectsSortIndex), TargetChainDirectionCalCulat/1(RE_StationaryObjectsSortIndex)
  Theta_Calculation/2(StillTarget12_0_Theta_ALL) -> RE_EgoRight2TargetTheta/1, Unit Delay1/1
  TargetChainDirectionCalCulat/1(RE_TargetChainStartDir) -> RE_EgoRightTargetChainStartDirection/1
  TargetChainDirectionCalCulat/2(RE_TargetChainDir) -> RE_EgoRightTargetChainDirection/1
  RE_EdgeElementID_K1/1 -> Dy_Filter/4(RE_EdgeElementID_K1)  "RE_EdgeElementID_K1"

== system PubIfDecisionTOS_MDL/TOS_20201112/TOS_2012080320/PP1128/AAT-AdditionalAttributes/RoadEdge/RE_2020_12_07/RoadEdge_V2/TargetChain/ObjectIsTargetChainElement ==
  note: 1、 目标链组成元素的计算判断；
      | 直向或者同向
      | A ：dx2-dx1 < 40m；
      | B ：dy2-dy1 < 3m；
      | 异向
      | A ：dx2-dx1 < 40m；
      | B ：dy2-dy1 < 1m；
      | 2、计算目标链个数
      | 3、计算目标链组成元素个数
  note: RE_TargetChainStartDir:
      |
      | 0:Invalid
      | 1:Stright Dir
      | 2:Left Dir
      | 3:Right Dir
  note: RE_TargetChainDir:
      |
      | 0:Invalid
      | 1:Stright_Same Dir
      | 2:Stright_Different Dir
      | 3:Left_Same Dir
      | 4:Left_Different Dir
      | 5:Right_Same Dir
      | 6:Right_Different Dir
  RE_EgoLeftTargetChainStartDirection : Inport  PortDimensions=80  BusOutputAsStruct=on
  RE_EgoLeftTargetChainDirection : Inport  Port=2  PortDimensions=80  BusOutputAsStruct=on
  RE_EgoLeftStill3TargetTheta : Inport  Port=3  OutDataTypeStr=single  PortDimensions=80  BusOutputAsStruct=on
  RE_EgoLeftStillTarget2Theta : Inport  Port=4  OutDataTypeStr=single  PortDimensions=80  BusOutputAsStruct=on
  OFM_Signal : Inport  Port=5  BusOutputAsStruct=on
  RE_EgoLeftStillObjectsSortIndex : Inport  Port=6  OutDataTypeStr=uint8  PortDimensions=80  BusOutputAsStruct=on
  RE_EgoRightStillObjectsSortIndex : Inport  Port=7  OutDataTypeStr=uint8  PortDimensions=80  BusOutputAsStruct=on
  RE_EgoRightTargetChainStartDirection : Inport  Port=8  PortDimensions=80  BusOutputAsStruct=on
  RE_EgoRightTargetChainDirection : Inport  Port=9  PortDimensions=80  BusOutputAsStruct=on
  RE_EgoRightStill3TargetTheta : Inport  Port=10  OutDataTypeStr=single  PortDimensions=80  BusOutputAsStruct=on
  RE_EgoRightStillTarget2Theta : Inport  Port=11  OutDataTypeStr=single  PortDimensions=80  BusOutputAsStruct=on
  Bus Creator : BusCreator  Inputs=11
  Bus Selector : BusSelector  OutputSignals=OFM_Signal.Object_DX,OFM_Signal.Object_DY,RE_EgoLeftStillObjectsSortIndex,RE_EgoLeftTargetChainDirection,RE_EgoLeftTargetChainStartDirection
  Bus Selector1 : BusSelector  OutputSignals=OFM_Signal.Object_DX,OFM_Signal.Object_DY,RE_EgoRightStillObjectsSortIndex,RE_EgoRightTargetChainDirection,RE_EgoRightTargetChainStartDirection
  Bus Selector2 : BusSelector  OutputSignals=RE_EgoLeftStill3TargetTheta,RE_EgoRightStill3TargetTheta,RE_EgoLeftStill2TargetTheta,RE_EgoRightStill2TargetTheta
  Bus Selector3 : BusSelector  OutputSignals=RE_EgoLeftStillObjectsSortIndex
  Bus Selector4 : BusSelector  OutputSignals=RE_EgoRightStillObjectsSortIndex
  EgoLeft_TargetChainElementJudge : Stateflow chart  TreatAsAtomicUnit=on
  EgoLeft_TargetChainInfor : Stateflow chart  TreatAsAtomicUnit=on
  EgoRight_TargetChainElementJudge : Stateflow chart  TreatAsAtomicUnit=on
  EgoRight_TargetChainInfor : Stateflow chart  TreatAsAtomicUnit=on
  Goto10 : Goto  Commented=on  GotoTag=RE_EgoRightTargetChainElementNum
  Goto4 : Goto  Commented=on  GotoTag=RE_EgoLeftTargetChainElementFlag
  Goto5 : Goto  Commented=on  GotoTag=RE_EgoLeftTargetChainElementCounter
  Goto6 : Goto  Commented=on  GotoTag=RE_EgoRightTargetChainElementCounter
  Goto8 : Goto  Commented=on  GotoTag=RE_EgoRightTargetChainElementFlag
  Goto9 : Goto  Commented=on  GotoTag=RE_EgoRightTargetChainIndex
  Terminator : Terminator
  Terminator1 : Terminator
  RE_EgoLeftTargetChainIndex : Outport
  RE_EgoLeftTargetChainElementNum : Outport  Port=2
  RE_EgoLeftTargetChainStartIndex : Outport  Port=3
  RE_EgoRightTargetChainIndex : Outport  Port=4
  RE_EgoRightTargetChainElementNum : Outport  Port=5
  RE_EgoRightTargetChainStartIndex : Outport  Port=6
  RE_EgoLeft3TargetTheta : Outport  Port=7
  RE_EgoRight3TargetTheta : Outport  Port=8
  RE_EgoLeft2TargetTheta : Outport  Port=9
  RE_EgoRight2TargetTheta : Outport  Port=10
  wires:
  RE_EgoLeftTargetChainDirection/1 -> Bus Creator/2  "RE_EgoLeftTargetChainDirection"
  RE_EgoRightTargetChainDirection/1 -> Bus Creator/5  "RE_EgoRightTargetChainDirection"
  OFM_Signal/1 -> Bus Creator/7  "OFM_Signal"
  Bus Creator/1 -> Bus Selector4/1, Bus Selector2/1, Bus Selector1/1, Bus Selector/1, Bus Selector3/1
  RE_EgoLeftStillObjectsSortIndex/1 -> [RE_EgoLeftStillObjectsSortIndex], Bus Creator/8  "RE_EgoLeftStillObjectsSortIndex"
  RE_EgoLeftTargetChainStartDirection/1 -> Bus Creator/1  "RE_EgoLeftTargetChainStartDirection"
  RE_EgoRightTargetChainStartDirection/1 -> Bus Creator/4  "RE_EgoRightTargetChainStartDirection"
  Bus Selector/1 -> EgoLeft_TargetChainElementJudge/1(Object_Dx)  "<Object_DX>"
  Bus Selector/2 -> EgoLeft_TargetChainElementJudge/2(Object_Dy)  "<Object_DY>"
  Bus Selector/3 -> EgoLeft_TargetChainElementJudge/3(RE_StationaryObjectsSortIndex)  "<RE_EgoLeftStillObjectsSortIndex>"
  Bus Selector/4 -> EgoLeft_TargetChainElementJudge/4(RE_TargetChainDirection)  "<RE_EgoLeftTargetChainDirection>"
  Bus Selector/5 -> EgoLeft_TargetChainElementJudge/5(RE_TargetChainStartDirection)  "<RE_EgoLeftTargetChainStartDirection>"
  Bus Selector1/5 -> EgoRight_TargetChainElementJudge/5(RE_TargetChainStartDirection)  "<RE_EgoRightTargetChainStartDirection>"
  Bus Selector1/4 -> EgoRight_TargetChainElementJudge/4(RE_TargetChainDirection)  "<RE_EgoRightTargetChainDirection>"
  Bus Selector1/3 -> EgoRight_TargetChainElementJudge/3(RE_StationaryObjectsSortIndex)  "<RE_EgoRightStillObjectsSortIndex>"
  Bus Selector1/1 -> EgoRight_TargetChainElementJudge/1(Object_Dx)  "<Object_DX>"
  Bus Selector1/2 -> EgoRight_TargetChainElementJudge/2(Object_Dy)  "<Object_DY>"
  EgoLeft_TargetChainInfor/1(TargetChainIndex) -> RE_EgoLeftTargetChainIndex/1, [RE_EgoLeftTargetChainIndex]
  EgoLeft_TargetChainInfor/2(TargetChainElementNum) -> RE_EgoLeftTargetChainElementNum/1, [RE_EgoLeftTargetChainElementNum]
  EgoLeft_TargetChainElementJudge/1(RE_TargetChainElementFlag) -> Goto4/1, Terminator/1
  EgoLeft_TargetChainElementJudge/2(TargetChainStartIndex) -> EgoLeft_TargetChainInfor/2(TargetChainStartIndex), [RE_EgoLeftTargetChainStartIndex]
  RE_EgoLeftStill3TargetTheta/1 -> Bus Creator/3  "RE_EgoLeftStill3TargetTheta"
  RE_EgoRightStill3TargetTheta/1 -> Bus Creator/6  "RE_EgoRightStill3TargetTheta"
  Bus Selector2/1 -> RE_EgoLeft3TargetTheta/1  "<RE_EgoLeftStill3TargetTheta>"
  Bus Selector2/2 -> RE_EgoRight3TargetTheta/1  "<RE_EgoRightStill3TargetTheta>"
  RE_EgoLeftStillTarget2Theta/1 -> Bus Creator/10  "RE_EgoLeftStill2TargetTheta"
  RE_EgoRightStillTarget2Theta/1 -> Bus Creator/11  "RE_EgoRightStill2TargetTheta"
  Bus Selector2/3 -> RE_EgoLeft2TargetTheta/1  "<RE_EgoLeftStill2TargetTheta>"
  Bus Selector2/4 -> RE_EgoRight2TargetTheta/1  "<RE_EgoRightStill2TargetTheta>"
  Bus Selector3/1 -> EgoLeft_TargetChainInfor/1(RE_StationaryObjectsSortIndex)  "<RE_EgoLeftStillObjectsSortIndex>"
  EgoLeft_TargetChainElementJudge/3(ElementCounter) -> Goto5/1, EgoLeft_TargetChainInfor/3(ElementCounter)
  EgoRight_TargetChainElementJudge/1(RE_TargetChainElementFlag) -> Goto8/1, Terminator1/1
  EgoRight_TargetChainElementJudge/2(TargetChainStartIndex) -> EgoRight_TargetChainInfor/2(TargetChainStartIndex), [RE_EgoRightTargetChainStartIndex]
  EgoRight_TargetChainInfor/1(TargetChainIndex) -> Goto9/1, RE_EgoRightTargetChainIndex/1
  Bus Selector4/1 -> EgoRight_TargetChainInfor/1(RE_StationaryObjectsSortIndex)  "<RE_EgoRightStillObjectsSortIndex>"
  EgoRight_TargetChainElementJudge/3(ElementCounter) -> EgoRight_TargetChainInfor/3(ElementCounter), Goto6/1
  [RE_EgoLeftTargetChainStartIndex] -> RE_EgoLeftTargetChainStartIndex/1
  [RE_EgoRightTargetChainStartIndex] -> RE_EgoRightTargetChainStartIndex/1
  EgoRight_TargetChainInfor/2(TargetChainElementNum) -> Goto10/1, RE_EgoRightTargetChainElementNum/1
  RE_EgoRightStillObjectsSortIndex/1 -> [RE_EgoRightStillObjectsSortIndex], Bus Creator/9  "RE_EgoRightStillObjectsSortIndex"
